simulink model "tanksPID"  (Simulink 7.0)
settings: Solver=ode5  StartTime=0.0  StopTime=300  FixedStep=0.1  RelTol=1e-3
libraries: simulink x1, simulink_extras x1
settings Model: Creator=Paul Acquatella  LastModifiedBy=Mey
settings DebuggingCC: SaveWithParameterizedLinksMsg=none  SignalResolutionControl=TryResolveAllWithWarning  SolverPrmCheckMsg=none  MultiTaskDSMMsg=warning  MultiTaskCondExecSysMsg=none  StrictBusMsg=None
settings HardwareCC: TargetEndianess=LittleEndian  TargetHWDeviceType=MATLAB Host  ProdEqTarget=off
settings RTWCC: IncludeERTFirstTime=on
settings GRTTargetCC: TargetFcnLib=ansi_tfl_tmw.mat

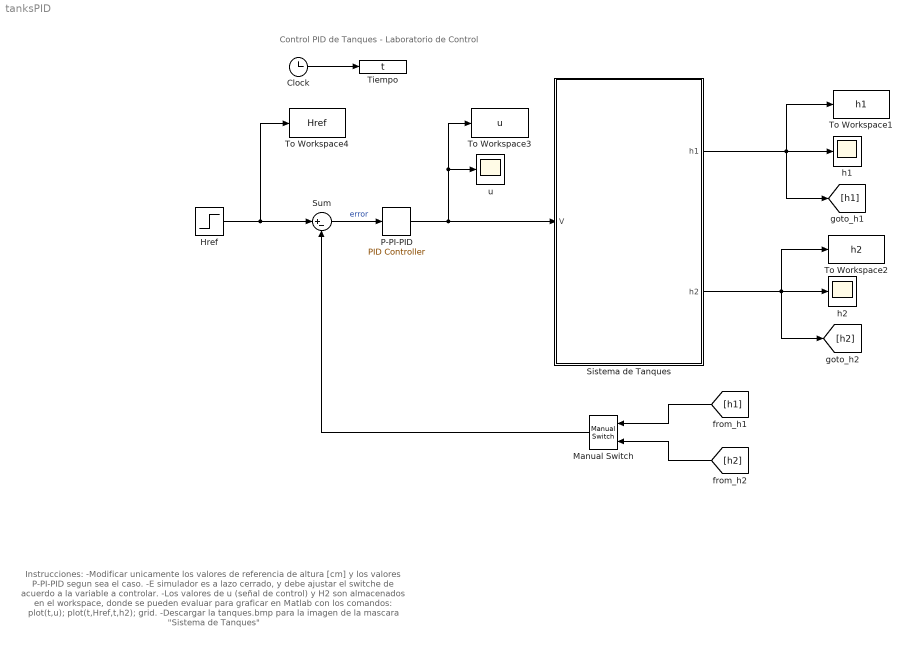
== system tanksPID ==
  note: Control PID de Tanques - Laboratorio de Control
  note: Instrucciones:
      | -Modificar unicamente los valores de referencia de altura [cm] y los valores P-PI-PID segun
      | sea el caso.
      | -E simulador es a lazo cerrado, y debe ajustar el switche de acuerdo a la variable
      | a controlar.
      | -Los valores de u (señal de control) y H2 son almacenados en el workspace, donde se pueden
      | evaluar para graficar en Matlab con los comandos: plot(t,u); plot(t,Href,t,h2); grid.
      | -Descargar la tanques.bmp para la imagen de la mascara "Sistema de Tanques"
  Clock : Clock
      settings: Decimation=10
  Href : Step  Time=110  Before=5.5  After=6.7
  Manual Switch : simulink/Signal Routing/Manual Switch  Orientation=left  SystemSampleTime=-1  sw=1  action=0  varsize=off
  P-PI-PID : simulink_extras/Additional Linear/PID Controller  SystemSampleTime=-1  P=16.62  I=3.08  D=22.437
  Sistema de Tanques : Subsystem
      mask Display: image(imread('tanques.bmp'))
  Sum : Sum  Inputs=|+-  OutDataType=sfix(16)  OutScaling=2^0
  Tiempo : ToWorkspace  VariableName=t  SaveFormat=Array
  To Workspace1 : ToWorkspace  VariableName=h1  SaveFormat=Array
  To Workspace2 : ToWorkspace  VariableName=h2  SaveFormat=Array
  To Workspace3 : ToWorkspace  VariableName=u  SaveFormat=Array
  To Workspace4 : ToWorkspace  VariableName=Href  SaveFormat=Array
  h1 : Scope
  h2 : Scope
  u : Scope
      settings: SaveName=ScopeData2
  wires:
  Clock/1 -> Tiempo/1
  Sistema de Tanques/1(h1) -> h1/1, To Workspace1/1, [h1]
  Sistema de Tanques/2(h2) -> To Workspace2/1, h2/1, [h2]
  Href/1 -> Sum/1, To Workspace4/1
  Sum/1 -> P-PI-PID/1  "error"
  P-PI-PID/1 -> Sistema de Tanques/1(V), To Workspace3/1, u/1
  [h1] -> Manual Switch/1
  [h2] -> Manual Switch/2
  Manual Switch/1 -> Sum/2

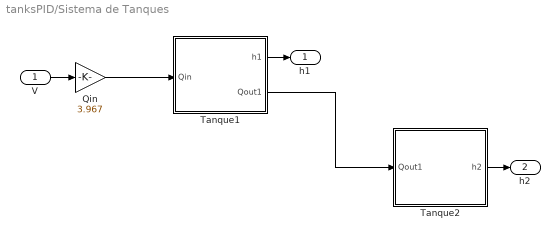
== system tanksPID/Sistema de Tanques ==
  V : Inport
  Qin : Gain  Gain=3.967  ParameterDataType=sfix(16)  ParameterScaling=2^0  OutDataType=sfix(16)  OutScaling=2^0
  Tanque1 : Subsystem
  Tanque2 : Subsystem
  h1 : Outport
  h2 : Outport  Port=2
  wires:
  Qin/1 -> Tanque1/1(Qin)
  Tanque1/2(Qout1) -> Tanque2/1(Qout1)
  Tanque1/1(h1) -> h1/1
  V/1 -> Qin/1
  Tanque2/1(h2) -> h2/1

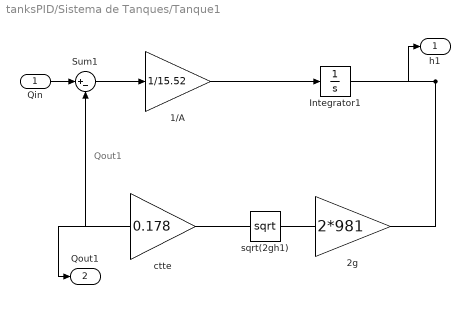
== system tanksPID/Sistema de Tanques/Tanque1 ==
  note: Qout1
  Qin : Inport  OutDataType=sfix(16)  OutScaling=2^0
  1/A : Gain  Gain=1/15.52  ParameterDataType=sfix(16)  ParameterScaling=2^0  OutDataType=sfix(16)  OutScaling=2^0
  2g : Gain  Gain=2*981  ParameterDataType=sfix(16)  ParameterScaling=2^0  OutDataType=sfix(16)  OutScaling=2^0
  Integrator1 : Integrator
  Sum1 : Sum  Inputs=|+-  OutDataType=sfix(16)  OutScaling=2^0  InputSameDT=on
  ctte : Gain  Gain=0.178  ParameterDataType=sfix(16)  ParameterScaling=2^0  OutDataType=sfix(16)  OutScaling=2^0
  sqrt(2gh1) : Math  Operator=sqrt  OutDataType=sfix(16)  OutScaling=2^0  SaturateOnIntegerOverflow=on
  h1 : Outport  OutDataType=sfix(16)  OutScaling=2^0
  Qout1 : Outport  Port=2  OutDataType=sfix(16)  OutScaling=2^0
  wires:
  2g/1 -> sqrt(2gh1)/1
  sqrt(2gh1)/1 -> ctte/1
  Sum1/1 -> 1/A/1
  1/A/1 -> Integrator1/1
  Integrator1/1 -> 2g/1, h1/1
  ctte/1 -> Sum1/2, Qout1/1
  Qin/1 -> Sum1/1

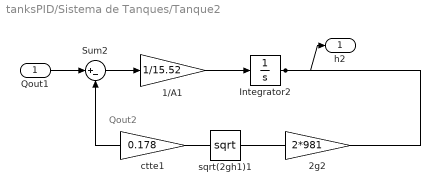
== system tanksPID/Sistema de Tanques/Tanque2 ==
  note: Qout2
  Qout1 : Inport  OutDataType=sfix(16)  OutScaling=2^0
  1/A1 : Gain  Gain=1/15.52  ParameterDataType=sfix(16)  ParameterScaling=2^0  OutDataType=sfix(16)  OutScaling=2^0
  2g2 : Gain  Gain=2*981  ParameterDataType=sfix(16)  ParameterScaling=2^0  OutDataType=sfix(16)  OutScaling=2^0
  Integrator2 : Integrator
  Sum2 : Sum  Inputs=|+-  OutDataType=sfix(16)  OutScaling=2^0  InputSameDT=on
  ctte1 : Gain  Gain=0.178  ParameterDataType=sfix(16)  ParameterScaling=2^0  OutDataType=sfix(16)  OutScaling=2^0
  sqrt(2gh1)1 : Math  Operator=sqrt  OutDataType=sfix(16)  OutScaling=2^0  SaturateOnIntegerOverflow=on
  h2 : Outport  OutDataType=sfix(16)  OutScaling=2^0
  wires:
  2g2/1 -> sqrt(2gh1)1/1
  sqrt(2gh1)1/1 -> ctte1/1
  ctte1/1 -> Sum2/2
  Sum2/1 -> 1/A1/1
  1/A1/1 -> Integrator2/1
  Integrator2/1 -> 2g2/1, h2/1
  Qout1/1 -> Sum2/1
